simulink model "ex5_1"  (R2020a)
settings: Solver=VariableStepAuto  StartTime=0.0  StopTime=10.0  RelTol=1e-3
libraries: simulink x2
settings Model: Creator=Kundan Patil  LastModifiedBy=Kundan Patil

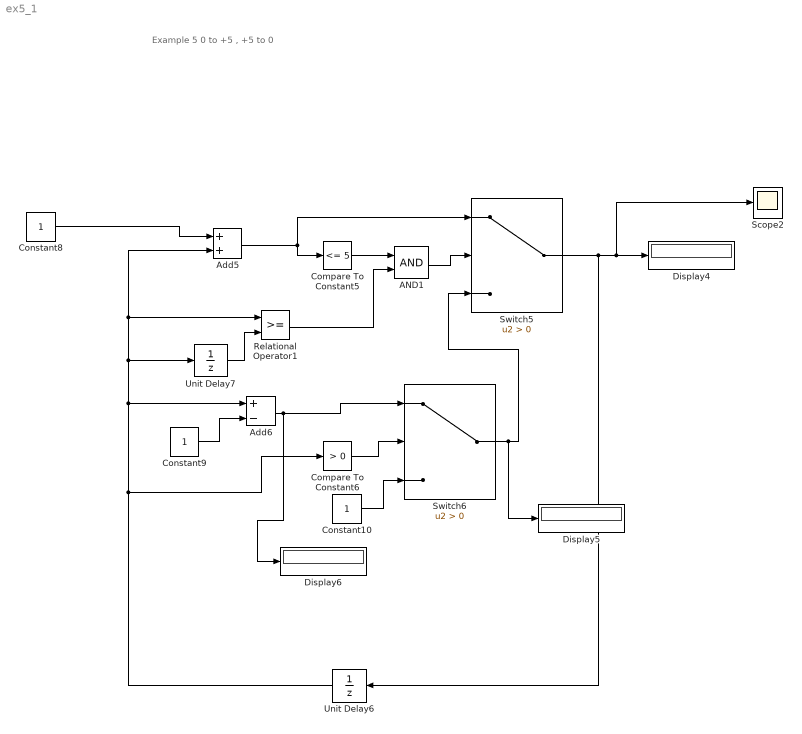
== system ex5_1 ==
  note: Example 5
      | 0 to +5 , +5 to  0
  AND1 : Logic  AllPortsSameDT=off  OutDataTypeStr=boolean
  Add5 : Sum
  Add6 : Sum  Inputs=+-
  Compare To Constant5 : simulink/Logic and Bit Operations/Compare To Constant  relop=<=  const=5  OutDataTypeStr=boolean
  Compare To Constant6 : simulink/Logic and Bit Operations/Compare To Constant  relop=>  const=0  OutDataTypeStr=boolean
  Constant10 : Constant
  Constant8 : Constant
  Constant9 : Constant
  Display4 : Display
  Display5 : Display
  Display6 : Display
  Relational Operator1 : RelationalOperator  OutDataTypeStr=boolean  RndMeth=Simplest
  Scope2 : Scope
  Switch5 : Switch  Criteria=u2 > Threshold
  Switch6 : Switch  Criteria=u2 > Threshold
  Unit Delay6 : UnitDelay  InitialCondition=-1  SampleTime=-1  HasFrameUpgradeWarning=on
  Unit Delay7 : UnitDelay  InitialCondition=-1  SampleTime=-1  HasFrameUpgradeWarning=on
  wires:
  Add6/1 -> Display6/1, Switch6/1
  Unit Delay7/1 -> Relational Operator1/2
  Switch6/1 -> Display5/1, Switch5/3
  Constant10/1 -> Switch6/3
  Relational Operator1/1 -> AND1/2
  Constant8/1 -> Add5/1
  Compare To Constant5/1 -> AND1/1
  Unit Delay6/1 -> Compare To Constant6/1, Relational Operator1/1, Add5/2, Unit Delay7/1, Add6/1
  Switch5/1 -> Unit Delay6/1, Scope2/1, Display4/1
  Compare To Constant6/1 -> Switch6/2
  Constant9/1 -> Add6/2
  Add5/1 -> Compare To Constant5/1, Switch5/1
  AND1/1 -> Switch5/2
